simulink model "PickPlaceWorkflowSimulinkMobileArm"  (R2022a)
settings: Solver=FixedStepAuto  StartTime=0.0  StopTime=Inf  FixedStep=Ts  RelTol=1e-3
model workspace (MAT data in the model file):
  SL_ROS_VariableLengthArrays_MaxSizes.CommonInfo.ArrayTruncateAction = 'EmitWarning'
  SL_ROS_VariableLengthArrays_MaxSizes.MsgTypeMap = containers.Map
  SL_ROS_VariableLengthArrays_MaxSizes.MsgTypeMap.serialization.keys = {'gazebo_msgs/ModelStates', 'sensor_msgs/Image', 'sensor_msgs/PointCloud2'}
  SL_ROS_VariableLengthArrays_MaxSizes.MsgTypeMap.serialization.values{1}(1).PropertyName = 'Name'
  SL_ROS_VariableLengthArrays_MaxSizes.MsgTypeMap.serialization.values{1}(1).DataType = 'std_msgs/String'
  SL_ROS_VariableLengthArrays_MaxSizes.MsgTypeMap.serialization.values{1}(1).MaxLength = 20
  SL_ROS_VariableLengthArrays_MaxSizes.MsgTypeMap.serialization.values{1}(2).PropertyName = 'Pose'
  SL_ROS_VariableLengthArrays_MaxSizes.MsgTypeMap.serialization.values{1}(2).DataType = 'geometry_msgs/Pose'
  SL_ROS_VariableLengthArrays_MaxSizes.MsgTypeMap.serialization.values{1}(2).MaxLength = 20
  SL_ROS_VariableLengthArrays_MaxSizes.MsgTypeMap.serialization.values{1}(3).PropertyName = 'Twist'
  SL_ROS_VariableLengthArrays_MaxSizes.MsgTypeMap.serialization.values{1}(3).DataType = 'geometry_msgs/Twist'
  SL_ROS_VariableLengthArrays_MaxSizes.MsgTypeMap.serialization.values{1}(3).MaxLength = 20
  SL_ROS_VariableLengthArrays_MaxSizes.MsgTypeMap.serialization.values{2}(1).PropertyName = 'Data'
  SL_ROS_VariableLengthArrays_MaxSizes.MsgTypeMap.serialization.values{2}(1).DataType = 'uint8'
  SL_ROS_VariableLengthArrays_MaxSizes.MsgTypeMap.serialization.values{2}(1).MaxLength = 518400
  SL_ROS_VariableLengthArrays_MaxSizes.MsgTypeMap.serialization.values{2}(2).PropertyName = 'Encoding'
  SL_ROS_VariableLengthArrays_MaxSizes.MsgTypeMap.serialization.values{2}(2).DataType = 'uint8'
  SL_ROS_VariableLengthArrays_MaxSizes.MsgTypeMap.serialization.values{2}(2).MaxLength = 128
  SL_ROS_VariableLengthArrays_MaxSizes.MsgTypeMap.serialization.values{3}(1).PropertyName = 'Data'
  SL_ROS_VariableLengthArrays_MaxSizes.MsgTypeMap.serialization.values{3}(1).DataType = 'uint8'
  SL_ROS_VariableLengthArrays_MaxSizes.MsgTypeMap.serialization.values{3}(1).MaxLength = 4147200
  SL_ROS_VariableLengthArrays_MaxSizes.MsgTypeMap.serialization.values{3}(2).PropertyName = 'Fields'
  SL_ROS_VariableLengthArrays_MaxSizes.MsgTypeMap.serialization.values{3}(2).DataType = 'sensor_msgs/PointField'
  SL_ROS_VariableLengthArrays_MaxSizes.MsgTypeMap.serialization.values{3}(2).MaxLength = 16
  SL_ROS_VariableLengthArrays_MaxSizes.MsgTypeMap.serialization.uniformity = 0
  SL_ROS_VariableLengthArrays_MaxSizes.MsgTypeMap.serialization.keyType = 'char'
  SL_ROS_VariableLengthArrays_MaxSizes.MsgTypeMap.serialization.valueType = 'any'
undefined symbols (not defined in the file or in its folder): Angular, detectionArmPose, eul2tform, gray, homeArmPose, homeRobotPose, Linear, logicalMap, placingArmPose, placingRobotPose1, placingRobotPose2, trvec2tform, Ts
libraries: robotlib x12, robotmaniplib x3, visionanalysis x1, robotcorelib x1, robotalgslib x1
settings Model: Creator=The MathWorks, Inc.  LastModifiedBy=The MathWorks, Inc.
settings SolverCC: AlgebraicLoopSolver=TrustRegion  MaxZcPerStep=1
settings OptimizationCC: EnhancedBackFolding=on  PassReuseOutputArgsAs=Individual arguments  ZeroExternalMemoryAtStartup=off  ZeroInternalMemoryAtStartup=off  MaxStackSize=64  OptimizeBlockOrder=speed  DifferentSizesBufferReuse=on  OptimizationCustomize=off  EfficientTunableParamExpr=on
settings DebuggingCC: ParameterTunabilityLossMsg=error  UnconnectedInputMsg=warning  UnconnectedOutputMsg=warning  UnconnectedLineMsg=warning  SFMachineParentedDataDiag=warning
settings HardwareCC: ProdBitPerPointer=32  ProdBitPerSizeT=32  ProdBitPerPtrDiffT=32  ProdLargestAtomicFloat=None  ProdIntDivRoundTo=Undefined  ProdEndianess=Unspecified  ProdWordSize=32  ProdHWDeviceType=Generic->Unspecified (assume 32-bit Generic)
settings SFSimCC: SimTargetLang=C++
settings RTWCC: SystemTargetFile=ert.tlc  HardwareBoard=Robot Operating System (ROS)  TLCOptions="-aInlineSetEventsForThisBaseRateFcn=TLC_FALSE -aSuppressMultiTaskScheduler=TLC_FALSE  -aRateBasedStepFcn=0"  TemplateMakefile=ert_default_tmf  Toolchain=Catkin  TargetLang=C++  DLArmComputeVersion=19.05
settings CodeAppCC: ForceParamTrailComments=on  IgnoreCustomStorageClasses=off  OperatorAnnotations=on  SimulinkDataObjDesc=on  SFDataObjDesc=on  InsertBlockDesc=on

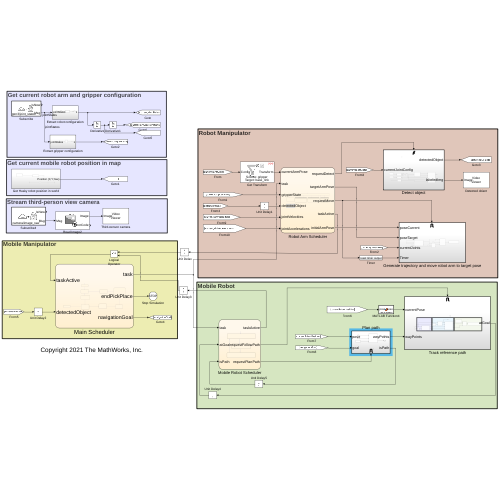
[thumbnail: Simulink's stored preview of the top-level diagram]
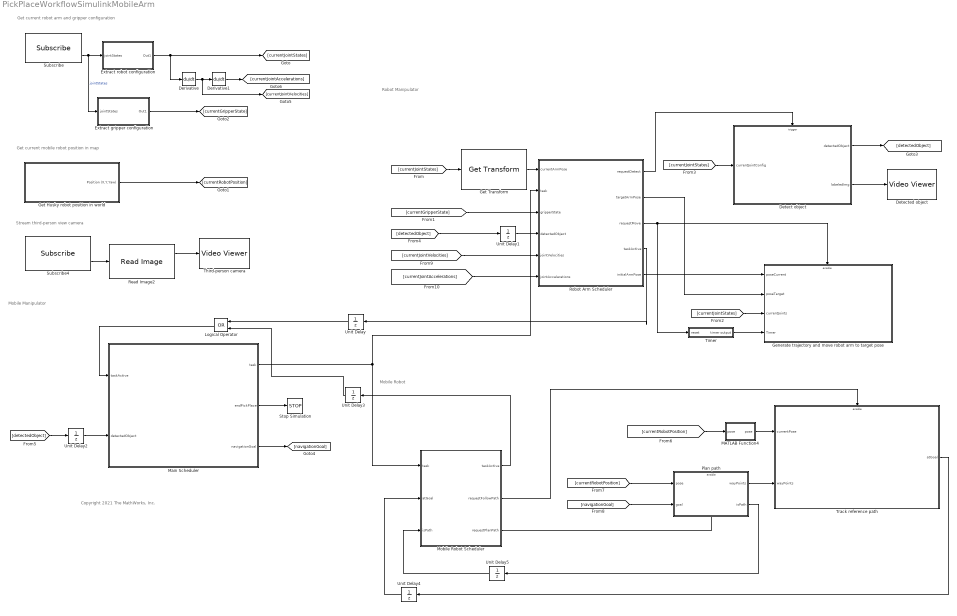
== system PickPlaceWorkflowSimulinkMobileArm ==
  note: Mobile Manipulator
  note: Mobile Robot
  note: Robot Manipulator
  note: Stream third-person view camera
  note: Get current mobile robot position in map
  note: Get current robot arm and gripper configuration
  note: Copyright 2021 The MathWorks, Inc.
  Derivative : Derivative
  Derivative1 : Derivative
  Detect object : Subsystem
  Detected object : VideoViewer  colormapValue=gray(256)  FigPos=[74 1091.33333333333 664.333333333333 562.333333333333]
  Extract gripper configuration : Subsystem
  Extract robot configuration : Subsystem
  Generate trajectory and move robot arm to target pose : Subsystem
  Get Husky robot position in world : Subsystem
  Get Transform : robotmaniplib/Get Transform  RigidBodyTree=robot  SourceBody=gripper  TargetBody=base_link  SimulateUsing=Code generation
  Logical Operator : Logic  Operator=OR  AllPortsSameDT=off  OutDataTypeStr=boolean
  MATLAB Function4 : MATLAB Function  TreatAsAtomicUnit=on
  Main Scheduler : Stateflow chart  TreatAsAtomicUnit=on
  Mobile Robot Scheduler : Stateflow chart  TreatAsAtomicUnit=on
  Plan path : Subsystem
  Read Image2 : robotlib/Read Image  MaximumImageSize=[270, 480]  ImageEncoding=rgb8  ShowAlphaOutput=off  ShowErrorCodeOutput=on  VariableSizeOutputs=off
      settings: SourceProductBaseCode=RR
  Robot Arm Scheduler : Stateflow chart  TreatAsAtomicUnit=on
  Stop Simulation : Stop
  Subscribe : robotlib/Subscribe  topicSource=Select from ROS network  topic=/husky_gen3/joint_states  messageType=sensor_msgs/JointState  SampleTime=-1  legacyBusStruct=off  messageQueueLength=1
  Subscribe4 : robotlib/Subscribe  topicSource=Select from ROS network  topic=/thirdperson_camera/image_raw  messageType=sensor_msgs/Image  SampleTime=-1  legacyBusStruct=off  messageQueueLength=1
  Third-person camera : VideoViewer  colormapValue=gray(256)  FigPos=[35 465.333333333333 579.333333333333 292]
  Timer : Subsystem
  Track reference path : Subsystem
  Unit Delay : UnitDelay  SampleTime=-1  HasFrameUpgradeWarning=on
  Unit Delay1 : UnitDelay  InitialCondition=[2,0,0,0,0]  SampleTime=-1  HasFrameUpgradeWarning=on
  Unit Delay2 : UnitDelay  InitialCondition=[2,0,0,0,0]  SampleTime=-1  HasFrameUpgradeWarning=on
  Unit Delay3 : UnitDelay  SampleTime=-1  HasFrameUpgradeWarning=on
  Unit Delay4 : UnitDelay  SampleTime=-1  HasFrameUpgradeWarning=on
  Unit Delay5 : UnitDelay  InitialCondition=false  SampleTime=-1  HasFrameUpgradeWarning=on
  wires:
  Robot Arm Scheduler/2(targetArmPose) -> Generate trajectory and move robot arm to target pose/2(poseTarget)
  Robot Arm Scheduler/3(requestMove) -> Generate trajectory and move robot arm to target pose/Enable, Timer/1(reset)
  Get Transform/1 -> Robot Arm Scheduler/1(currentArmPose)
  [currentJointStates] -> Get Transform/1
  [currentJointStates] -> Generate trajectory and move robot arm to target pose/3(currentJoints)
  Get Husky robot position in world/1(Position (X,Y,Yaw)) -> [currentRobotPosition]
  Robot Arm Scheduler/4(taskActive) -> Unit Delay/1
  Robot Arm Scheduler/1(requestDetect) -> Detect object/Trigger
  Detect object/2(labeledImg) -> Detected object/1
  [currentJointStates] -> Detect object/1(currentJointConfig)
  Subscribe/2 -> Extract robot configuration/1(jointStates), Extract gripper configuration/1(jointStates)  "jointStates"
  Extract gripper configuration/1(Out1) -> [currentGripperState]
  Extract robot configuration/1(Out1) -> Derivative/1, [currentJointStates]
  [currentGripperState] -> Robot Arm Scheduler/3(gripperState)
  Detect object/1(detectedObject) -> [detectedObject]
  Unit Delay1/1 -> Robot Arm Scheduler/4(detectedObject)
  [detectedObject] -> Unit Delay1/1
  Unit Delay2/1 -> Main Scheduler/2(detectedObject)
  [detectedObject] -> Unit Delay2/1
  Main Scheduler/2(endPickPlace) -> Stop Simulation/1
  Mobile Robot Scheduler/1(taskActive) -> Unit Delay3/1
  Unit Delay/1 -> Logical Operator/1
  Unit Delay3/1 -> Logical Operator/2
  Logical Operator/1 -> Main Scheduler/1(taskActive)
  [navigationGoal] -> Plan path/2(goal)
  MATLAB Function4/1(pose) -> Track reference path/1(currentPose)
  Plan path/1(wayPoints) -> Track reference path/2(wayPoints)
  [currentRobotPosition] -> MATLAB Function4/1("pose ")
  Track reference path/1(atGoal) -> Unit Delay4/1
  Mobile Robot Scheduler/3(requestPlanPath) -> Plan path/Enable
  [currentRobotPosition] -> Plan path/1(pose)
  Main Scheduler/3(navigationGoal) -> [navigationGoal]
  Unit Delay4/1 -> Mobile Robot Scheduler/2(atGoal)
  Mobile Robot Scheduler/2(requestFollowPath) -> Track reference path/Enable
  Plan path/2(isPath) -> Unit Delay5/1
  Unit Delay5/1 -> Mobile Robot Scheduler/3(isPath)
  Subscribe4/2 -> Read Image2/1
  Read Image2/1 -> Third-person camera/1
  Derivative/1 -> [currentJointVelocities], Derivative1/1
  Derivative1/1 -> [currentJointAccelerations]
  [currentJointVelocities] -> Robot Arm Scheduler/5(jointVelocities)
  [currentJointAccelerations] -> Robot Arm Scheduler/6(jointAccelerations)
  Robot Arm Scheduler/5(initialArmPose) -> Generate trajectory and move robot arm to target pose/1(poseCurrent)
  Timer/1(timer output) -> Generate trajectory and move robot arm to target pose/4(Timer)
  Main Scheduler/1(task) -> Mobile Robot Scheduler/1(task), Robot Arm Scheduler/2(task)

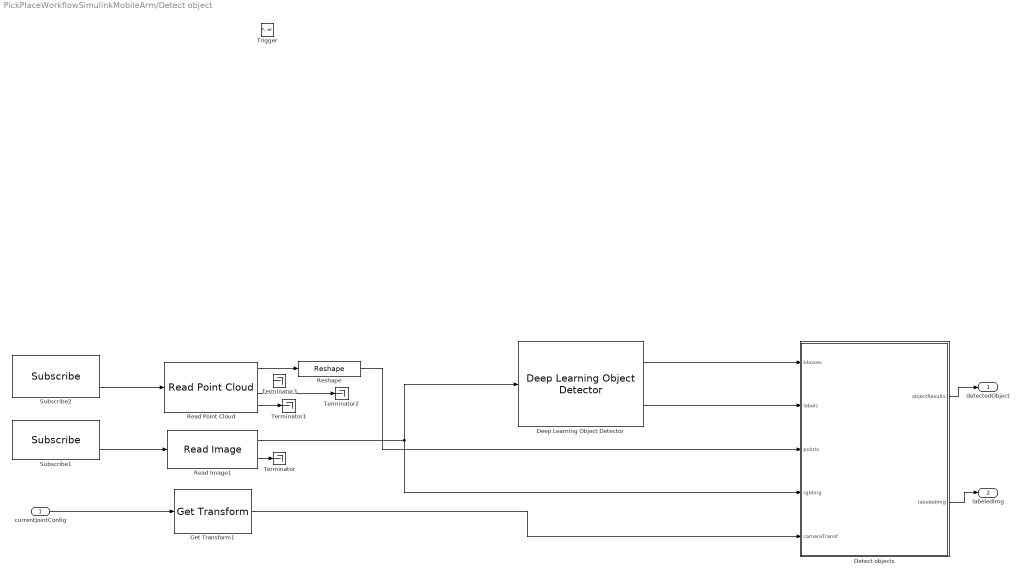
== system PickPlaceWorkflowSimulinkMobileArm/Detect object ==
  currentJointConfig : Inport
  Trigger : TriggerPort  VariantControl=Variant  PortDimensions=1
  Deep Learning Object Detector : visionanalysis/Deep Learning Object Detector  Detector=Detector from MAT-file  DetectorFunction=untitled  DetectorFilePath=helperYolo2DetectorMobileArm.mat  MaxDetections=500  Bboxes=on  Scores=off  UseROI=off  ROI=[1 1 100 100]  Threshold=0.5  NumStrongestRegions=2000  UseMinSize=off  MinSize=[1 1]  UseMaxSize=off  MaxSize=[50 50]  ForceInterpretedSim=off
      settings: SourceProductBaseCode=VP
  Detect objects : MATLAB Function  TreatAsAtomicUnit=on
  Get Transform1 : robotmaniplib/Get Transform  RigidBodyTree=robot  SourceBody=EndEffector_Link  TargetBody=base_link  SimulateUsing=Interpreted execution
  Read Image1 : robotlib/Read Image  MaximumImageSize=[270, 480]  ImageEncoding=rgb8  ShowAlphaOutput=off  ShowErrorCodeOutput=on  VariableSizeOutputs=off
      settings: SourceProductBaseCode=RR
  Read Point Cloud : robotlib/Read Point Cloud  MaximumPointCloudSize=[270, 480]  PreserveStructure=off  ShowRGBOutput=on  ShowIntensityOutput=on  ShowErrorCodeOutput=on  VariableSizeOutputs=off
      settings: SourceProductBaseCode=RR
  Reshape : Reshape  OutputDimensionality=Customize  OutputDimensions=[480, 270 ,3]
  Subscribe1 : robotlib/Subscribe  topicSource=Select from ROS network  topic=/camera/color/image_raw  messageType=sensor_msgs/Image  SampleTime=-1  legacyBusStruct=off  messageQueueLength=1
  Subscribe2 : robotlib/Subscribe  topicSource=Select from ROS network  topic=/camera/depth/points  messageType=sensor_msgs/PointCloud2  SampleTime=-1  legacyBusStruct=off  messageQueueLength=1
  Terminator{,1..3} (4 alike) : Terminator
  detectedObject : Outport
  labeledImg : Outport  Port=2
  wires:
  Subscribe1/2 -> Read Image1/1
  currentJointConfig/1 -> Get Transform1/1
  Read Image1/1 -> Deep Learning Object Detector/1, Detect objects/4(rgbImg)
  Read Point Cloud/1 -> Reshape/1
  Subscribe2/2 -> Read Point Cloud/1
  Detect objects/2(labeledImg) -> labeledImg/1
  Detect objects/1(objectResults) -> detectedObject/1
  Reshape/1 -> Detect objects/3(points)
  Get Transform1/1 -> Detect objects/5(cameraTransf)
  Read Image1/2 -> Terminator/1
  Read Point Cloud/3 -> Terminator2/1
  Read Point Cloud/4 -> Terminator1/1
  Deep Learning Object Detector/1 -> Detect objects/1(bboxes)
  Deep Learning Object Detector/2 -> Detect objects/2(labels)

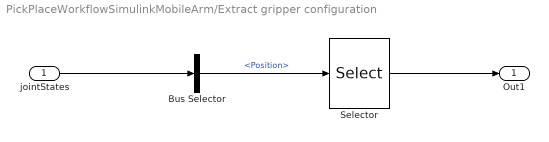
== system PickPlaceWorkflowSimulinkMobileArm/Extract gripper configuration ==
  jointStates : Inport
  Bus Selector : BusSelector  OutputSignals=Position
  Selector : Selector  InputPortWidth=128  IndexOptions=Index vector (dialog)  Indices=3  OutputSizes=1
  Out1 : Outport
  wires:
  jointStates/1 -> Bus Selector/1
  Selector/1 -> Out1/1
  Bus Selector/1 -> Selector/1  "<Position>"

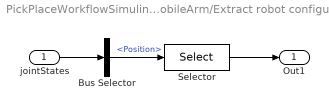
== system PickPlaceWorkflowSimulinkMobileArm/Extract robot configuration ==
  jointStates : Inport
  Bus Selector : BusSelector  OutputSignals=Position
  Selector : Selector  InputPortWidth=128  IndexOptions=Index vector (dialog)  Indices=[4:10]  OutputSizes=1
  Out1 : Outport
  wires:
  Bus Selector/1 -> Selector/1  "<Position>"
  jointStates/1 -> Bus Selector/1
  Selector/1 -> Out1/1

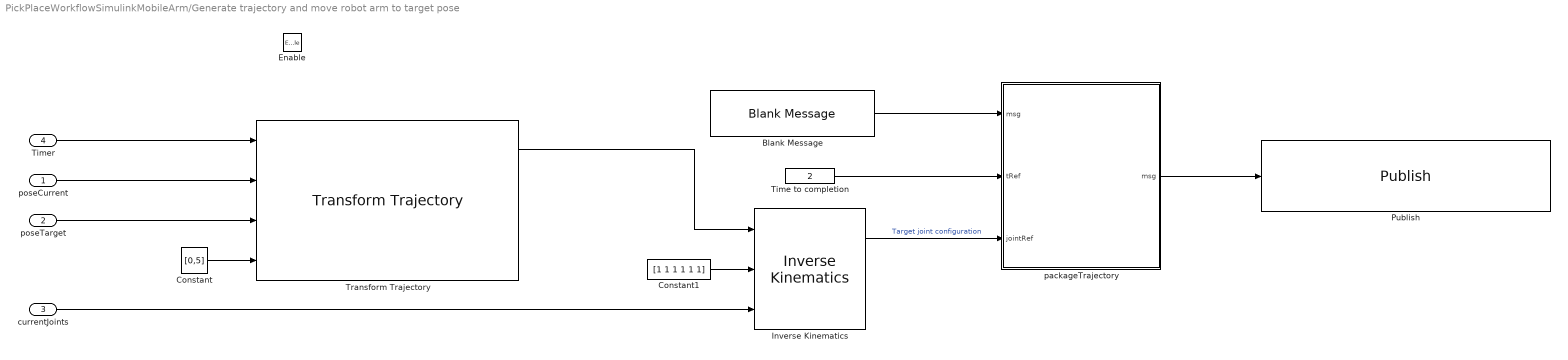
== system PickPlaceWorkflowSimulinkMobileArm/Generate trajectory and move robot arm to target pose ==
  poseCurrent : Inport
  poseTarget : Inport  Port=2
  currentJoints : Inport  Port=3
  Timer : Inport  Port=4
  Enable : EnablePort
  Blank Message : robotlib/Blank Message  messageClass=Message  entityType=trajectory_msgs/JointTrajectory  messageType=trajectory_msgs/JointTrajectory  SampleTime=inf  legacyBusStruct=off
  Constant : Constant  Value=[0,5]  VectorParams1D=off  SampleTime=Ts
  Constant1 : Constant  Value=[1 1 1 1 1 1]
  Inverse Kinematics : robotmaniplib/Inverse Kinematics  RigidBodyTree=robot  EndEffector=gripper  ShowInfo=on  SolverName=BFGS Gradient Projection  EnforceJointLimits=off  MaxIterations=1500  MaxTime=10  GradientTolerance=1e-7  SolutionTolerance=1e-6  StepTolerance=1e-14  ErrorChangeTolerance=1e-12  UseErrorDamping=on  DampingBias=0.0025  SimulateUsing=Code generation
  Publish : robotlib/Publish  topicSource=Select from ROS network  topic=/husky_gen3/gen3_joint_trajectory_controller/command  messageType=trajectory_msgs/JointTrajectory  legacyBusStruct=off  messageQueueLength=1
  Time to completion : Constant  Value=2
  Transform Trajectory : robotcorelib/Transform Trajectory  WaypointSource=External  T0=trvec2tform( [ 1, 10, -1 ] )  TF=eul2tform( [ 0, pi, pi / 2 ] )  TimeInterval=[ 2, 3 ]  CustomTimeScaling=off  ParameterSource=Internal  TSTime=2:0.1:3  TimeScaling=[ 0:0.1:1; ones( 1, 11 ); zeros( 1, 11 ) ]  SimulateUsing=Code generation
      settings: SourceProductBaseCode=RO,NV,RR,UV
  packageTrajectory : MATLAB Function  TreatAsAtomicUnit=on
  wires:
  Constant1/1 -> Inverse Kinematics/2
  Inverse Kinematics/1 -> packageTrajectory/3(jointRef)  "Target joint configuration"
  Transform Trajectory/1 -> Inverse Kinematics/1
  Time to completion/1 -> packageTrajectory/2(tRef)
  currentJoints/1 -> Inverse Kinematics/3
  Constant/1 -> Transform Trajectory/4
  poseTarget/1 -> Transform Trajectory/3
  poseCurrent/1 -> Transform Trajectory/2
  Blank Message/1 -> packageTrajectory/1("msg ")
  Timer/1 -> Transform Trajectory/1
  packageTrajectory/1(msg) -> Publish/1

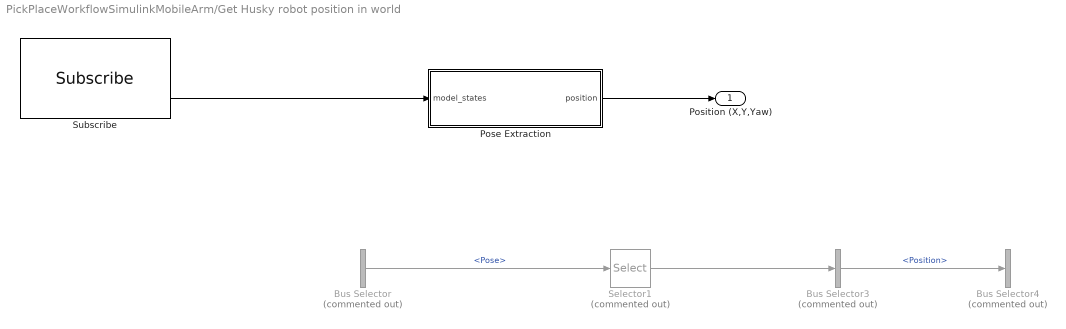
== system PickPlaceWorkflowSimulinkMobileArm/Get Husky robot position in world ==
  Bus Selector : BusSelector  Commented=on  OutputSignals=Pose
  Bus Selector3 : BusSelector  Commented=on  OutputSignals=Position
  Bus Selector4 : BusSelector  Commented=on  OutputSignals=X
  Pose Extraction : MATLAB Function  TreatAsAtomicUnit=on
  Selector1 : Selector  Commented=on  InputPortWidth=16  IndexOptions=Index vector (dialog)  Indices=12  OutputSizes=1
  Subscribe : robotlib/Subscribe  topicSource=Select from ROS network  topic=/gazebo/model_states  messageType=gazebo_msgs/ModelStates  SampleTime=-1  legacyBusStruct=off  messageQueueLength=1
  Position (X,Y,Yaw) : Outport  VectorParamsAs1DForOutWhenUnconnected=off
  wires:
  Subscribe/2 -> Pose Extraction/1(model_states)
  Bus Selector/1 -> Selector1/1  "<Pose>"
  Selector1/1 -> Bus Selector3/1
  Bus Selector3/1 -> Bus Selector4/1  "<Position>"
  Pose Extraction/1(position) -> Position (X,Y,Yaw)/1

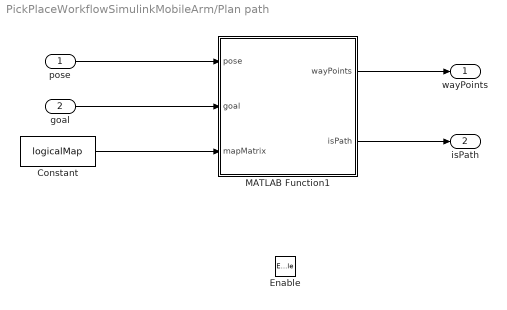
== system PickPlaceWorkflowSimulinkMobileArm/Plan path ==
  pose : Inport
  goal : Inport  Port=2
  Enable : EnablePort  PropagateVarSize=During execution
  Constant : Constant  Value=logicalMap
  MATLAB Function1 : MATLAB Function  TreatAsAtomicUnit=on
  wayPoints : Outport
  isPath : Outport  Port=2
  wires:
  pose/1 -> MATLAB Function1/1(pose)
  goal/1 -> MATLAB Function1/2(goal)
  MATLAB Function1/1(wayPoints) -> wayPoints/1
  Constant/1 -> MATLAB Function1/3(mapMatrix)
  MATLAB Function1/2(isPath) -> isPath/1

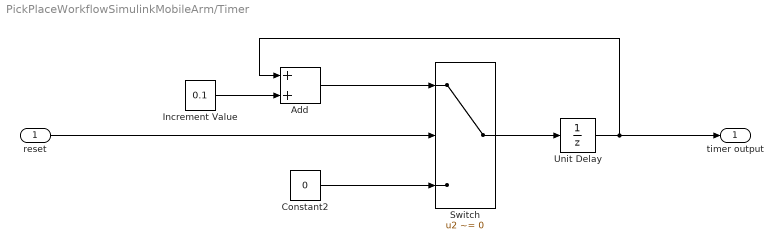
== system PickPlaceWorkflowSimulinkMobileArm/Timer ==
  reset : Inport
  Add : Sum
  Constant2 : Constant  Value=0
  Increment Value : Constant  Value=0.1  SampleTime=Ts
  Switch : Switch  Criteria=u2 ~= 0  SaturateOnIntegerOverflow=off  InputSameDT=off
  Unit Delay : UnitDelay  SampleTime=-1  HasFrameUpgradeWarning=on
  timer output : Outport
  wires:
  Add/1 -> Switch/1
  Switch/1 -> Unit Delay/1
  reset/1 -> Switch/2
  Unit Delay/1 -> timer output/1, Add/1
  Increment Value/1 -> Add/2
  Constant2/1 -> Switch/3

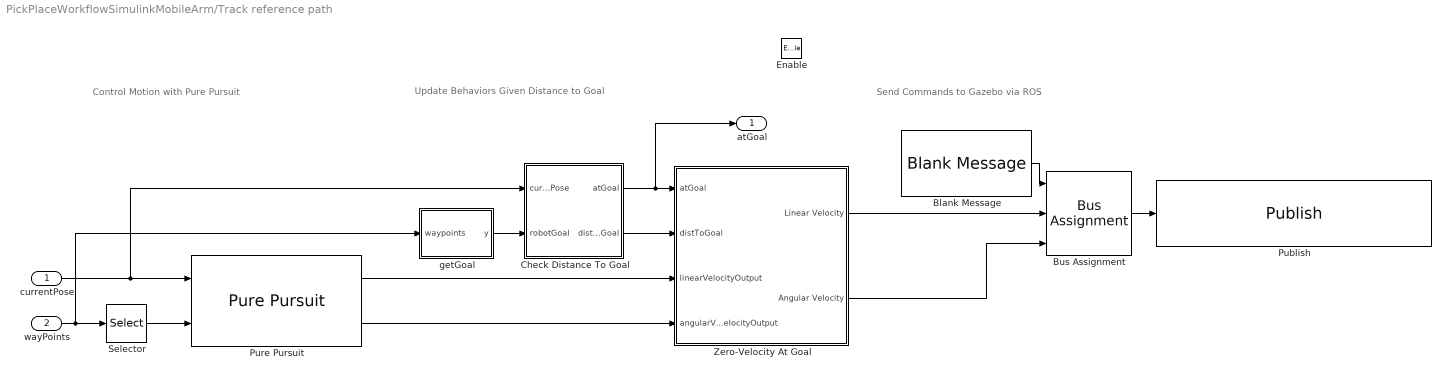
== system PickPlaceWorkflowSimulinkMobileArm/Track reference path ==
  note: Control Motion with Pure Pursuit
  note: Send Commands to Gazebo via ROS
  note: Update Behaviors Given Distance to Goal
  currentPose : Inport
  wayPoints : Inport  Port=2
  Enable : EnablePort
  Blank Message : robotlib/Blank Message  messageClass=Message  entityType=geometry_msgs/Twist  messageType=geometry_msgs/Twist  SampleTime=0  legacyBusStruct=off
  Bus Assignment : BusAssignment  DialogController=Simulink.DDGSource_BusAssignment  AssignedSignals=Linear.X,Angular.Z
  Check Distance To Goal : Subsystem
  Publish : robotlib/Publish  topicSource=Select from ROS network  topic=/husky_gen3/husky_velocity_controller/cmd_vel  messageType=geometry_msgs/Twist  legacyBusStruct=off  messageQueueLength=105
  Pure Pursuit : robotalgslib/Pure Pursuit  DesiredLinearVelocity=1.0  MaxAngularVelocity=1.2  LookaheadDistance=0.7  TargetDirPort=off  SimulateUsing=Code generation
  Selector : Selector  NumberOfDimensions=2  InputPortWidth=3  IndexOptions=Select all,Index vector (dialog)  Indices=[1 2],[1 2]  OutputSizes=1,1
  Zero-Velocity At Goal : Subsystem
  getGoal : MATLAB Function  TreatAsAtomicUnit=on
  atGoal : Outport
  wires:
  Pure Pursuit/2 -> Zero-Velocity At Goal/4(angularVelocityOutput)
  wayPoints/1 -> getGoal/1(waypoints), Selector/1
  currentPose/1 -> Pure Pursuit/1, Check Distance To Goal/1(currentPose)
  Bus Assignment/1 -> Publish/1
  Blank Message/1 -> Bus Assignment/1
  Check Distance To Goal/1(atGoal) -> atGoal/1, Zero-Velocity At Goal/1(atGoal)
  Selector/1 -> Pure Pursuit/2
  getGoal/1(y) -> Check Distance To Goal/2(robotGoal)
  Zero-Velocity At Goal/1(Linear Velocity) -> Bus Assignment/2
  Zero-Velocity At Goal/2(Angular Velocity) -> Bus Assignment/3
  Pure Pursuit/1 -> Zero-Velocity At Goal/3(linearVelocityOutput)
  Check Distance To Goal/2(distToGoal) -> Zero-Velocity At Goal/2(distToGoal)

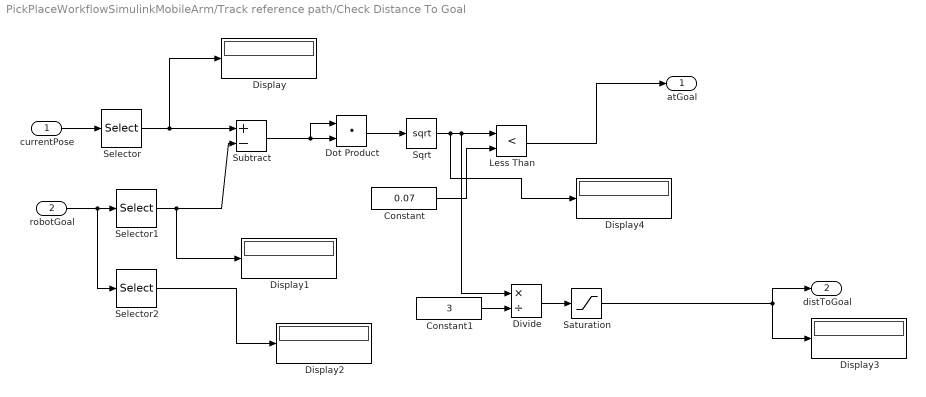
== system PickPlaceWorkflowSimulinkMobileArm/Track reference path/Check Distance To Goal ==
  currentPose : Inport
  robotGoal : Inport  Port=2
  Constant : Constant  Value=0.07
  Constant1 : Constant  Value=3
  Display{,1..4} (5 alike) : Display
  Divide : Product  Inputs=*/
  Dot Product : DotProduct  OutDataTypeStr=Inherit: Inherit via internal rule
  Less Than : RelationalOperator  Operator=<  OutDataTypeStr=boolean  RndMeth=Simplest  InputSameDT=off
  Saturation : Saturate  UpperLimit=1  LowerLimit=0.2
  Selector : Selector  InputPortWidth=3  IndexOptions=Index vector (dialog)  Indices=[1 2]  OutputSizes=1
  Selector1 : Selector  InputPortWidth=3  IndexOptions=Index vector (dialog)  Indices=[1 2]  OutputSizes=1
  Selector2 : Selector  InputPortWidth=3  IndexOptions=Index vector (dialog)  Indices=3  OutputSizes=1
  Sqrt : Sqrt
  Subtract : Sum  Inputs=+-
  atGoal : Outport
  distToGoal : Outport  Port=2
  wires:
  robotGoal/1 -> Selector2/1, Selector1/1
  Dot Product/1 -> Sqrt/1
  Constant/1 -> Less Than/2
  currentPose/1 -> Selector/1
  Sqrt/1 -> Display4/1, Divide/1, Less Than/1
  Subtract/1 -> Dot Product/1, Dot Product/2
  Selector/1 -> Display/1, Subtract/1
  Selector1/1 -> Subtract/2, Display1/1
  Selector2/1 -> Display2/1
  Less Than/1 -> atGoal/1
  Saturation/1 -> distToGoal/1, Display3/1
  Constant1/1 -> Divide/2
  Divide/1 -> Saturation/1

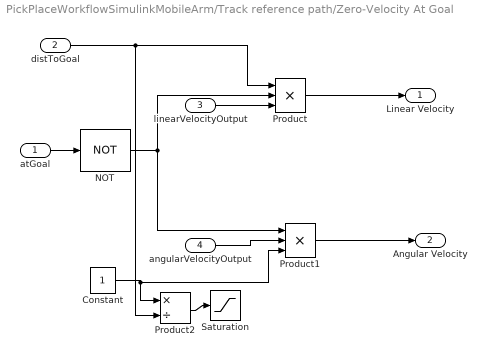
== system PickPlaceWorkflowSimulinkMobileArm/Track reference path/Zero-Velocity At Goal ==
  atGoal : Inport
  distToGoal : Inport  Port=2
  linearVelocityOutput : Inport  Port=3
  angularVelocityOutput : Inport  Port=4
  Constant : Constant  VectorParams1D=off  SampleTime=-1
  NOT : Logic  Operator=NOT  IconShape=distinctive  AllPortsSameDT=off  OutDataTypeStr=boolean
  Product : Product  Inputs=3
  Product1 : Product  Inputs=3
  Product2 : Product  Inputs=*/
  Saturation : Saturate  UpperLimit=1.5  LowerLimit=1
  Linear Velocity : Outport  OutDataTypeStr=double
  Angular Velocity : Outport  Port=2  OutDataTypeStr=double
  wires:
  atGoal/1 -> NOT/1
  angularVelocityOutput/1 -> Product1/2
  linearVelocityOutput/1 -> Product/3
  Product/1 -> Linear Velocity/1
  Product1/1 -> Angular Velocity/1
  NOT/1 -> Product1/1, Product/2
  distToGoal/1 -> Product2/2, Product/1
  Constant/1 -> Product1/3, Product2/1
  Product2/1 -> Saturation/1

== matlab function PickPlaceWorkflowSimulinkMobileArm/Detect object/Detect objects ==
  data: bboxes input; labels input; points input; rgbImg input; objectResults output; cameraTransf input; labeledImg output
function [objectResults,labeledImg] = detectObjects(bboxes, labels, points, rgbImg, cameraTransf)

% Copyright 2021 The MathWorks, Inc.

    % Initialization
    objectLocation = [0,0,0];
    objectDetected = 0;
    objectType = 0;
    objectResults = [objectDetected, objectLocation, objectType];
    labeledImg = rgbImg;

    % As long as there is labeled data, proceed
    if ~isempty(labels)
        % The object detector returns an array of labels, which in Simulink
        % are treated as enums, meaning they can be evaluated using an
        % integer. To see which enumeration equates to which label, call
        % the following on the command line after updating (Ctrl+D) the
        % model:
        %    helperYolo2DetectorMobileArm_labels(1)
        %    helperYolo2DetectorMobileArm_labels(2)
        %  These return enumerations for "bottle_label" and "can_label",
        %  respectively. Hence in this function, instead of comparing to
        %  the string (which is also possible), we will check if the label
        %  is equal to 1 for the bottle and 2 for the can.

        % Label the image using the data from the object detector block
        for j = 1:numel(labels)
            labeledImg = insertObjectAnnotation(labeledImg,'Rectangle',bboxes(j,:),{char(labels(j))}); 
        end
        
        % If there is more than one detected object and the first item is a
        % can, start with the bottle (i.e. the second item)
        labelIdx=1;
        if labels(labelIdx)==2 && numel(labels)>1
            labelIdx = 2;
        end
        
        % Determine the object type: 1 for the can and 2 for the bottle. It
        % would be easier if this matched the labels, but this requires
        % some downstream changes.
        if labels(labelIdx)==2
            objectType = 1; % Can
        else 
            objectType = 2; % Bottle
        end
        
        % Camera is misaligned wrt end-effector link
        eeToCamera = [1.0000    0.0000    0.0000    0.0000; ...
                      0.0000   -1.0000    0.0000    0.0550;...
                      0.0000   -0.0000   -1.0000   -0.0065;...
                      0         0         0    1.0000];
                  
        eeToRealee = [1.0000    0.0000   -0.0000   -0.0000;...
                     -0.0000    1.0000    0.0000    0.0000;...
                      0.0000   -0.0000    1.0000    0.0020;...
                      0         0         0    1.0000];
                  
        actualCameraTransf = cameraTransf * eeToRealee * eeToCamera; %trvec2tform([0, 0.055, -0.005]); 
        
        % Center pixel of detected object
        centerBox = [bboxes(labelIdx,2) + round(bboxes(labelIdx,4)/2), bboxes(labelIdx,1)+ round(bboxes(labelIdx,3)/2)];
        
        % Object pose wrt camera frame      
        partZ = double(points(centerBox(2),centerBox(1),3));
        partX = double(points(centerBox(2),centerBox(1),2));
        partY = double(points(centerBox(2),centerBox(1),1));
        
        % Object pose wrt robot base frame
        centerpointTransf = actualCameraTransf * trvec2tform([-partY,partX,-partZ]);
        centerPoint = centerpointTransf(1:3,4)';
        
        % Store and output results
        objectLocation = centerPoint;
        objectDetected = 1;
        objectResults = [objectDetected, objectLocation, objectType];
     end
end

== stateflow chart PickPlaceWorkflowSimulinkMobileArm/Main Scheduler ==
  state Start
    en:
    task = Tasks.Idle;
    taskActiveLocal = taskActive;
  state NavigateToPlacingPose
    en, du:
    if detectedObject(5)==2
    navigationGoal = placingRobotPose1;
    else
    navigationGoal = placingRobotPose2;
    end
    task = Tasks.Robot_Navigate;
    exit: task = Tasks.Idle;
  state PlaceObject
    en, du:
    task = Tasks.Arm_Place;
    exit: task = Tasks.Idle;
  state MoveArmHome
    en, du:
    task = Tasks.Arm_Home;
    exit: task = Tasks.Idle;
  state NavigateToHomePose
    en, du:
    navigationGoal = homeRobotPose;;
    task = Tasks.Robot_Navigate;
    exit: task = Tasks.Idle;
  state PickObject
    en:
    task = Tasks.Arm_Pick;
    taskActiveLocal = true;
    during:
    taskActiveLocal = taskActive;
    task = Tasks.Arm_Pick;
  state DetectObject
    en, du: task = Tasks.Arm_Detect;
    exit: task = Tasks.Idle;
  state MoveArmHome1
    en, du:
    task = Tasks.Arm_Home;
    exit: task = Tasks.Idle;
  state End1
    en,du:
    task = Tasks.Idle;
    endPickPlace = 1;
  note: No object was detected
  note: Object was detected
  (default) -> Start
  Start -> MoveArmHome : [taskActive==false]
  NavigateToPlacingPose -> PlaceObject : [taskActive==false]
  PlaceObject -> MoveArmHome : [taskActive==false]
  MoveArmHome -> NavigateToHomePose : [taskActive==false]
  MoveArmHome1 -> NavigateToPlacingPose : [taskActive==false]
  NavigateToHomePose -> DetectObject : [taskActive==false]
  DetectObject -> PickObject [order 1] : [taskActive==false && detectedObject(1)==1]
  DetectObject -> End1 [order 2] : [taskActive==false && detectedObject(1)==0]
  PickObject -> MoveArmHome1 : [taskActive==false]
  data: task output Enum: Tasks; taskActive input boolean; detectedObject input; endPickPlace output =0; placingRobotPose1 parameter; placingRobotPose2 parameter; navigationGoal output; homeRobotPose parameter; taskActiveLocal local boolean =false

== stateflow chart PickPlaceWorkflowSimulinkMobileArm/Robot Arm Scheduler ==
  state Idle
    en, du:
    requestMove = 0;
    requestDetect = 0;
    taskActive = false;
    initialArmPose = currentArmPose;
  state MoveToHome
    en:
    % Move to the robot's home configuration
    initialArmPose = currentArmPose;
    targetArmPose = homeArmPose;
    requestMove = 1;
    taskActive = true;
    success = false;
    during:
    success = goalReached(currentArmPose, targetArmPose, 0.1);
  state Detect
    state MoveToDetectionPose
      en:
      % Move to the robot's home configuration
      initialArmPose = currentArmPose;
      targetArmPose = detectionArmPose * trvec2tform(detectionPoseGrid*[0.15 0  0]);
      requestMove = 1;
      taskActive = true;
      success = false;
      during:
      success = goalReached(currentArmPose, targetArmPose, 0.02);
    note: A new object was detected or no object was detected after 4 attempts
    state Wait4
    note: No new object was detected at this pose
    state DetectObject1
      en:
      requestMove = 0;
      taskActive = true;
      requestDetect = 1; % send rising signal to request the Detection module to start running
      objectStatus = 2; % initialize objectStatus to show attempt to detect has not ended yet
      failedAttempts = failedAttempts + 1; % if an object is not detected the first time, try until you reach 3 failed attempts
      if detectionPoseGrid == 0
      detectionPoseGrid = -1;
      else
      detectionPoseGrid = -detectionPoseGrid;
      end
      during:
      requestDetect = 0;
      objectStatus = detectedObject(1); % update objectStatus based on input from the Detect module
    DetectObject1 -> MoveToDetectionPose [order 2] : [objectStatus==0 && failedAttempts<=4]
    MoveToDetectionPose -> Detect.Wait4 : [success==true]
    Detect.Wait4 -> DetectObject1 : after(1,sec)
  state PickObject
    state ApproachToPick
      % Approach detected object to pick from above
      en:
      taskActive = true;
      graspPose = computeGraspPose();  % compute grasp pose based on the location of detected object
      initialArmPose = currentArmPose;
      targetArmPose = graspPose * trvec2tform([0,0, -0.08]); % move to location above the object
      requestMove = 1;
      success = false;
      during:
      requestMove = 1;
      success = goalReached(currentArmPose, targetArmPose, 0.03);
    note: Robot has approached picking position
    state MoveToPick
      en:
      initialArmPose = currentArmPose;
      targetArmPose =  graspPose; % move to grasp pose
      requestMove = 1;
      during:
      requestMove = 1;
      success = goalReached(currentArmPose, targetArmPose, 0.01);
    state Wait3
    note: Robot has moved to picking position
    state CloseGripper
      en:
      activateGripper(1);
      during:
      activateGripper(1);
    state Wait2
    note: Robot has closed the gripper
    state PickUpObject
      initialArmPose = currentArmPose;
      targetArmPose =  graspPose * trvec2tform([0,0, -0.08]); % move to location above the object
      requestMove = 1;
      during:
      requestMove = 1;
      success = goalReached(currentArmPose, targetArmPose, 0.03);
    state BringObjectClose
      initialArmPose = currentArmPose;
      targetArmPose =  graspPose * trvec2tform([0,0, -0.05])* trvec2tform([0.2,0, 0]); % move to location above the object
      requestMove = 1;
      during:
      requestMove = 1;
      success = goalReached(currentArmPose, targetArmPose, 0.05);
    ApproachToPick -> MoveToPick : [success==true]{success = false; requestMove = 0}
    MoveToPick -> PickObject.Wait3 : [success==true]{success=false; requestMove =0}
    PickObject.Wait3 -> CloseGripper : after(1.0,sec)
    CloseGripper -> Wait2 : [gripperState>0.005]
    Wait2 -> PickUpObject : after(0.5,sec)
    PickUpObject -> BringObjectClose : [success==true]{success = false; requestMove = 0}
  state PlaceObject
    state MoveToPrePlacingPose1
      en:
      % Move to the robot's home configuration
      initialArmPose = currentArmPose;
      targetArmPose =trvec2tform([0.0 -0.6 0.4])*axang2tform([0 0 1 -pi/2])*axang2tform([0 1 0 pi/2]);
      requestMove = 1;
      taskActive = true;
      success = false;
      during:
      success = goalReached(currentArmPose, targetArmPose, 0.15);
    state MoveToPlacingPose
      en:
      % Move to the robot's home configuration
      initialArmPose = currentArmPose;
      targetArmPose = placingArmPose;
      requestMove = 1;
      taskActive = true;
      success = false;
      during:
      success = goalReached(currentArmPose, targetArmPose, 0.2);
    state Wait3
    state OpenGripper
      en:
      activateGripper(0);
      during:
      activateGripper(0);
    state MoveToPrePlacingPose2
      en:
      % Move to the robot's home configuration
      initialArmPose = currentArmPose;
      targetArmPose = trvec2tform([0.0 -0.6 0.4])*axang2tform([0 0 1 -pi/2])*axang2tform([0 1 0 pi/2]);
      requestMove = 1;
      taskActive = true;
      success = false;
      during:
      success = goalReached(currentArmPose, targetArmPose, 0.15);
    state Wait4
    MoveToPrePlacingPose1 -> MoveToPlacingPose : [success==true]{success=false; requestMove = 0}
    MoveToPlacingPose -> PlaceObject.Wait3 : [success==true]{success=false; requestMove = 0}
    PlaceObject.Wait3 -> OpenGripper : after(1,sec)
    OpenGripper -> MoveToPrePlacingPose2 : [gripperState<0.007]
    MoveToPrePlacingPose2 -> PlaceObject.Wait4 : [success==true]{success=false; requestMove = 0}
  PlaceObject.Wait4 -> Idle : after(0.5,sec)
  Idle -> ApproachToPick [order 2] : [task==Tasks.Arm_Pick]{taskActive = true;}
  DetectObject1 -> Idle [order 1] : [(objectStatus==1)||(objectStatus==0 ...
      |  && failedAttempts>4)]...
      | {failedAttempts = 0; objectStatus = 2}
  Idle -> MoveToDetectionPose [order 3] : [task==Tasks.Arm_Detect]{detectionPoseGrid = 0; failedAttempts = 0;}
  (default) -> Idle
  MoveToHome -> Idle : [success==true]
  Idle -> MoveToHome [order 1] : [task==Tasks.Arm_Home]
  Idle -> MoveToPrePlacingPose1 [order 4] : [task == Tasks.Arm_Place]
  BringObjectClose -> Idle : [success==true]{success=false; requestMove =0}
  data: taskCurrentLocal function_input; taskTargetLocal function_input; tolerance function_input; successLocal function_output; state function_input; graspPoseLocal function_output; requestDetect output =0; targetArmPose output =zeros(4,4); homeArmPose parameter; currentArmPose input; success local boolean =false; task input Enum: Tasks; requestMove output =0; taskActive output boolean; detectionArmPose parameter; gripperState input; failedAttempts local; detectedObject input; objectStatus local; graspPose local; placingArmPose parameter; detectionPoseGrid local; jointVelocities input; jointAccelerations input; initialArmPose output
  function successLocal = goalReached(taskCurrentLocal, taskTargetLocal, tolerance):
    | function successLocal = goalReached(taskCurrentLocal, taskTargetLocal, tolerance)
    |     successLocal = false;
    |     
    |     anglesTarget = rotm2quat(taskTargetLocal(1:3,1:3));
    |     poseTargetLocal = [taskTargetLocal(1:3,4);anglesTarget']; 
    |     anglesCurrent = rotm2quat(taskCurrentLocal(1:3,1:3));
    |     poseCurrentLocal =  [taskCurrentLocal(1:3,4);anglesCurrent'];
    |     angleDiff = quatmultiply(quatconj(anglesTarget), anglesCurrent);
    |     diffCurrent = abs([poseTargetLocal(1:3)-poseCurrentLocal(1:3); angleDiff(2:4)']);
    |     if all(abs(poseTargetLocal(1:3)-poseCurrentLocal(1:3))<tolerance) && abs(abs(angleDiff(1))-1)<0.01   
    |             successLocal = true; % goal achieved 
    |     end 
    |     
    | end
  function activateGripper(state):
    | function activateGripper(state)
    |   coder.extrinsic('helperActivateGripperMobileArm')
    |   helperActivateGripperMobileArm(state)
    | end
  function graspPoseLocal = computeGraspPose:
    | function graspPoseLocal = computeGraspPose()
    | 
    | detectedObjectLocal = detectedObject;
    | graspPoseLocal =  trvec2tform(detectedObjectLocal(2:4)' + [0 0 -0.035])*axang2tform([0 1 0 pi]);
    | 
    | % detectedObjectLocal(2) = detectedObject(3);
    | % detectedObjectLocal(3) = -detectedObject(2);
    | % graspPoseLocal = axang2tform([0 0 1 pi/2]) *  trvec2tform(detectedObjectLocal(2:4)' + [0 0 -0.04])*axang2tform([0 1 0 -pi]);
    | 
    | end

== matlab function PickPlaceWorkflowSimulinkMobileArm/Generate trajectory and move robot arm to target pose/packageTrajectory ==
  data: msg output; msg input Bus: SL_Bus_PickPlaceWorkflowSimulink_JointTrajectory_ezj767; tRef input; jointRef input
function msg = packageTrajectory(msg,tRef,jointRef)

%   This function packages the joint positions, velocities, and
%   accelerations of the desired trajectory into ROS messages as required
%   by ros_control

% Copyright 2021 The MathWorks, Inc.

    % Package joint names
    jointNames = {'joint_1','joint_2','joint_3','joint_4','joint_5','joint_6','joint_7'};
    numJoints = uint32(numel(jointNames));

    msg.JointNames_SL_Info.CurrentLength = uint32(7);
    for idx = 1:numJoints
       msg.JointNames(idx).Data(1:7) = uint8(jointNames{idx});
       msg.JointNames(idx).Data_SL_Info.CurrentLength = uint32(numJoints);
    end

    % Send next trajectory point
    msg.Points_SL_Info.CurrentLength = uint32(1);

    msg.Points(1).TimeFromStart.Sec = floor(tRef);
    msg.Points(1).TimeFromStart.Nsec = (tRef - floor(tRef))*1e9;

    msg.Points(1).Positions_SL_Info.CurrentLength = numJoints;
    msg.Points(1).Positions(1:numJoints) = jointRef;
    msg.Points(1).Velocities_SL_Info.CurrentLength = numJoints;
    msg.Points(1).Velocities(1:numJoints) = zeros(numJoints,1);
    msg.Points(1).Accelerations_SL_Info.CurrentLength = numJoints;
    msg.Points(1).Accelerations(1:numJoints) = zeros(numJoints,1);
    msg.Points(1).Effort_SL_Info.CurrentLength = numJoints;
    msg.Points(1).Effort(1:numJoints) = zeros(numJoints,1);
end

== matlab function PickPlaceWorkflowSimulinkMobileArm/Get Husky robot position in world/Pose Extraction ==
  data: model_states input; position output
function position = extractPose(model_states)

persistent huskyIdx

if isempty(huskyIdx)
    huskyIdx = 1;
    for msgIdx = 1:numel(model_states.Name)
        modelName = char(model_states.Name(msgIdx).Data');
        isHusky = contains(modelName,'husky_gen3');
        if isHusky
            huskyIdx = msgIdx;
            break
        end
    end
end

X = model_states.Pose(huskyIdx).Position.X;
Y = model_states.Pose(huskyIdx).Position.Y;
Xo = model_states.Pose(huskyIdx).Orientation.X;
Yo = model_states.Pose(huskyIdx).Orientation.Y;
Zo = model_states.Pose(huskyIdx).Orientation.Z;
Wo = model_states.Pose(huskyIdx).Orientation.W;

eul = quat2eul([Wo,Xo,Yo,Zo]);
yaw = eul(1);

position = [X,Y,yaw];
end

== stateflow chart PickPlaceWorkflowSimulinkMobileArm/Mobile Robot Scheduler ==
  state Idle
    en, du:
    requestPlanPath = 0;
    requestFollowPath= 0;
    taskActive = false;
  state PlanPath
    en:
    taskActive = true;
    requestPlanPath = 1;
  state FollowPath
    en:
    requestFollowPath = 1
    during:
    requestFollowPath = 1;
  (default) -> Idle
  FollowPath -> Idle : [atGoal == 1]
  Idle -> PlanPath : [task==Tasks.Robot_Navigate]
  PlanPath -> FollowPath : [isPath == true]{requestPlanPath = 0}
  data: task input Enum: Tasks; taskActive output boolean; atGoal input; isPath input boolean; requestFollowPath output; requestPlanPath output

== matlab function PickPlaceWorkflowSimulinkMobileArm/Plan path/MATLAB Function1 ==
  data: pose input size=[1 3]; goal input size=[1 3]; mapMatrix input; wayPoints output size=[1000 3]; isPath output boolean
function [wayPoints, isPath] = plan(pose,goal,mapMatrix)

% Copyright 2021 The MathWorks, Inc.

coder.extrinsic('helperPlotPathMobileArm');

ss = stateSpaceDubins; 

%Create an occupanyMap-based state validator using the created state space.
binaryMap = binaryOccupancyMap(mapMatrix,10);
sv = validatorOccupancyMap(ss,"Map",binaryMap);
startPose = pose;
endPose = goal;
isPath = false;

% check if start pose is sufficiently close to goal pose
orientationDif = abs(angdiff(startPose(3), endPose(3)));
positionDif = norm(startPose(1:2)-endPose(1:2)); 

if orientationDif<=0.1 && positionDif<=0.1
    wayPoints = startPose;
    isPath = true;
    helperPlotPathMobileArm(startPose,wayPoints, mapMatrix)
    return;
end




%Set validation distance for the validator.
sv.ValidationDistance = 0.05;%0.01
ss.StateBounds = [binaryMap.XWorldLimits;binaryMap.YWorldLimits; [-pi pi]];
ss.MinTurningRadius = 3;%1.5;
planner = plannerRRTStar(ss,sv);
planner.MaxConnectionDistance = 0.2; 
planner.MaxNumTreeNodes = 100000;

%Set the start and goal states.
planner.MaxIterations = 100000;
planner.GoalBias = 0.5;

disp('Planning path')

rng(1); % for repeatable result
[pthObj,solnInfo] = plan(planner,startPose,endPose);
isPath = solnInfo.IsPathFound;
%Visualize the results.
if isPath
    interpolate(pthObj, pthObj.NumStates * 2);
end
wayPoints = [pthObj.States;endPose]; 
helperPlotPathMobileArm(startPose,wayPoints, mapMatrix)

== matlab function PickPlaceWorkflowSimulinkMobileArm/MATLAB Function4 ==
  data: pose input; pose output
function pose = removeNan(pose)

if any(isnan(pose))
    pose = [1 1 0];
end

end

== matlab function PickPlaceWorkflowSimulinkMobileArm/Track reference path/getGoal ==
  data: waypoints input size=[1000 3]; y output double size=[1 3]
function y = getGoal(waypoints)
y = [0 0 0];
if ~isempty(waypoints)
    y = waypoints(end,1:3);
end
end
